simulink model "case9"  (R2024b)
settings: Solver=FixedStepAuto  StartTime=0  StopTime=1  FixedStep=1e-7  RelTol=1e-3
values from neighbouring files (symbols this model uses):
  SG_D_1_D = 0.01056    [IEEE9_case_parameters.m]    (also in case1_parameters.m; case2_parameters.m; case3_parameters.m; case4_parameters.m)
  SG_D_1_EnableSaturation = 0    [IEEE9_case_parameters.m]    (also in case1_parameters.m; case2_parameters.m; case3_parameters.m; case4_parameters.m)
  SG_D_1_f0 = 60    [IEEE9_case_parameters.m]    (also in case1_parameters.m; case2_parameters.m; case3_parameters.m; case4_parameters.m)
  SG_D_1_H = 7.5    [IEEE9_case_parameters.m]    (also in case1_parameters.m; case2_parameters.m; case3_parameters.m; case4_parameters.m)
  SG_D_1_K_A = 20    [IEEE9_case_parameters.m]    (also in case1_parameters.m; case2_parameters.m; case3_parameters.m; case4_parameters.m)
  SG_D_1_K_E = 1.000000e+1    (= 10)    [IEEE9_case_parameters.m]    (also in case1_parameters.m; case2_parameters.m; case3_parameters.m; case4_parameters.m)
  SG_D_1_K_F = 2.363    [IEEE9_case_parameters.m]    (also in case1_parameters.m; case2_parameters.m; case3_parameters.m; case4_parameters.m)
  SG_D_1_K_s = 0.5    [IEEE9_case_parameters.m]    (also in case1_parameters.m = 5; case2_parameters.m = 5; case3_parameters.m = 5; case4_parameters.m = 5)
  SG_D_1_R_a = 0.001088    [IEEE9_case_parameters.m]    (also in case1_parameters.m; case2_parameters.m; case3_parameters.m; case4_parameters.m)
  SG_D_1_S_A = 1    [IEEE9_case_parameters.m]    (also in case1_parameters.m; case2_parameters.m; case3_parameters.m; case4_parameters.m)
  SG_D_1_S_B = 0.103    [IEEE9_case_parameters.m]    (also in case1_parameters.m; case2_parameters.m; case3_parameters.m; case4_parameters.m)
  SG_D_1_S_N = 10.659857    [IEEE9_case_parameters.m]    (also in case1_parameters.m; case2_parameters.m; case3_parameters.m; case4_parameters.m)
  SG_D_1_SpeedPara = 200    [IEEE9_case_parameters.m]    (also in case1_parameters.m; case2_parameters.m; case3_parameters.m; case4_parameters.m)
  SG_D_1_T_0 = 0.720173    [IEEE9_case_parameters.m]    (also in case1_parameters.m = 0.755522; case2_parameters.m = 0.808931; case3_parameters.m = 0.869402; case4_parameters.m = 0.729316)
  SG_D_1_T_1 = 0.3    [IEEE9_case_parameters.m]    (also in case1_parameters.m; case2_parameters.m; case3_parameters.m; case4_parameters.m)
  SG_D_1_T_2 = 0.05    [IEEE9_case_parameters.m]    (also in case1_parameters.m; case2_parameters.m; case3_parameters.m; case4_parameters.m)
  SG_D_1_T_3 = 0.02    [IEEE9_case_parameters.m]    (also in case1_parameters.m; case2_parameters.m; case3_parameters.m; case4_parameters.m)
  SG_D_1_T_4 = 0.005    [IEEE9_case_parameters.m]    (also in case1_parameters.m; case2_parameters.m; case3_parameters.m; case4_parameters.m)
  SG_D_1_T_A = 0.02    [IEEE9_case_parameters.m]    (also in case1_parameters.m; case2_parameters.m; case3_parameters.m; case4_parameters.m)
  SG_D_1_T_dd = 8.000000e+0    (= 8)    [IEEE9_case_parameters.m]    (also in case1_parameters.m; case2_parameters.m; case3_parameters.m; case4_parameters.m)
  SG_D_1_T_ddd = 0.04    [IEEE9_case_parameters.m]    (also in case1_parameters.m; case2_parameters.m; case3_parameters.m; case4_parameters.m)
  SG_D_1_T_E = 0.314    [IEEE9_case_parameters.m]    (also in case1_parameters.m; case2_parameters.m; case3_parameters.m; case4_parameters.m)
  SG_D_1_T_F = 0.35    [IEEE9_case_parameters.m]    (also in case1_parameters.m; case2_parameters.m; case3_parameters.m; case4_parameters.m)
  SG_D_1_T_qd = 0.8    [IEEE9_case_parameters.m]    (also in case1_parameters.m; case2_parameters.m; case3_parameters.m; case4_parameters.m)
  SG_D_1_T_qdd = 0.02    [IEEE9_case_parameters.m]    (also in case1_parameters.m; case2_parameters.m; case3_parameters.m; case4_parameters.m)
  SG_D_1_T_speed = 0.1    [IEEE9_case_parameters.m]    (also in case1_parameters.m = 200; case2_parameters.m = 200; case3_parameters.m = 200; case4_parameters.m = 200)
  SG_D_1_T_w = 0.5    [IEEE9_case_parameters.m]    (also in case1_parameters.m; case2_parameters.m; case3_parameters.m; case4_parameters.m)
  SG_D_1_V_ref = 1.990276    [IEEE9_case_parameters.m]    (also in case1_parameters.m = 2.042296; case2_parameters.m = 2.051388; case3_parameters.m = 2.089584; case4_parameters.m = 2.01845)
  SG_D_1_w_ref = 376.991118    [IEEE9_case_parameters.m]    (also in case1_parameters.m; case2_parameters.m; case3_parameters.m; case4_parameters.m)
  SG_D_1_wb = 6.000000e+1    (= 60)    [IEEE9_case_parameters.m]    (also in case1_parameters.m; case2_parameters.m; case3_parameters.m; case4_parameters.m)
  SG_D_1_x_d = 1.9    [IEEE9_case_parameters.m]    (also in case1_parameters.m; case2_parameters.m; case3_parameters.m; case4_parameters.m)
  SG_D_1_x_dd = 0.302    [IEEE9_case_parameters.m]    (also in case1_parameters.m; case2_parameters.m; case3_parameters.m; case4_parameters.m)
  SG_D_1_x_ddd = 0.204    [IEEE9_case_parameters.m]    (also in case1_parameters.m; case2_parameters.m; case3_parameters.m; case4_parameters.m)
  SG_D_1_x_l = 0.05    [IEEE9_case_parameters.m]    (also in case1_parameters.m; case2_parameters.m; case3_parameters.m; case4_parameters.m)
  SG_D_1_x_q = 1.3    [IEEE9_case_parameters.m]    (also in case1_parameters.m; case2_parameters.m; case3_parameters.m; case4_parameters.m)
  SG_D_1_x_qd = 0.5    [IEEE9_case_parameters.m]    (also in case1_parameters.m; case2_parameters.m; case3_parameters.m; case4_parameters.m)
  SG_D_1_x_qdd = 0.3    [IEEE9_case_parameters.m]    (also in case1_parameters.m; case2_parameters.m; case3_parameters.m; case4_parameters.m)
  SG_D_2_D = 0.02    [IEEE9_case_parameters.m]    (also in case1_parameters.m; case2_parameters.m; case3_parameters.m; case4_parameters.m)
  SG_D_2_EnableSaturation = 0    [IEEE9_case_parameters.m]    (also in case1_parameters.m; case2_parameters.m; case3_parameters.m; case4_parameters.m)
  SG_D_2_f0 = 60    [IEEE9_case_parameters.m]    (also in case1_parameters.m; case2_parameters.m; case3_parameters.m; case4_parameters.m)
  SG_D_2_H = 8.000000e+0    (= 8)    [IEEE9_case_parameters.m]    (also in case1_parameters.m; case2_parameters.m; case3_parameters.m; case4_parameters.m)
  SG_D_2_K_A = 20    [IEEE9_case_parameters.m]    (also in case1_parameters.m; case2_parameters.m; case3_parameters.m; case4_parameters.m)
  SG_D_2_K_E = 1.000000e+1    (= 10)    [IEEE9_case_parameters.m]    (also in case1_parameters.m; case2_parameters.m; case3_parameters.m; case4_parameters.m)
  SG_D_2_K_F = 2.363    [IEEE9_case_parameters.m]    (also in case1_parameters.m; case2_parameters.m; case3_parameters.m; case4_parameters.m)
  SG_D_2_K_s = 0.5    [IEEE9_case_parameters.m]    (also in case1_parameters.m = 4; case2_parameters.m = 4; case3_parameters.m = 4; case4_parameters.m = 4)
  SG_D_2_R_a = 0.001088    [IEEE9_case_parameters.m]    (also in case1_parameters.m; case2_parameters.m; case3_parameters.m; case4_parameters.m)
  SG_D_2_S_A = 1    [IEEE9_case_parameters.m]    (also in case1_parameters.m; case2_parameters.m; case3_parameters.m; case4_parameters.m)
  SG_D_2_S_B = 0.103    [IEEE9_case_parameters.m]    (also in case1_parameters.m; case2_parameters.m; case3_parameters.m; case4_parameters.m)
  SG_D_2_S_N = 10.659857    [IEEE9_case_parameters.m]    (also in case1_parameters.m; case2_parameters.m; case3_parameters.m; case4_parameters.m)
  SG_D_2_SpeedPara = 200    [IEEE9_case_parameters.m]    (also in case1_parameters.m; case2_parameters.m; case3_parameters.m; case4_parameters.m)
  SG_D_2_T_0 = 1.632913    [IEEE9_case_parameters.m]    (also in case1_parameters.m = 1.632925; case2_parameters.m = 1.632915; case3_parameters.m = 1.632914; case4_parameters.m = 1.632927)
  SG_D_2_T_1 = 0.2    [IEEE9_case_parameters.m]    (also in case1_parameters.m; case2_parameters.m; case3_parameters.m; case4_parameters.m)
  SG_D_2_T_2 = 0.05    [IEEE9_case_parameters.m]    (also in case1_parameters.m; case2_parameters.m; case3_parameters.m; case4_parameters.m)
  SG_D_2_T_3 = 0.02    [IEEE9_case_parameters.m]    (also in case1_parameters.m; case2_parameters.m; case3_parameters.m; case4_parameters.m)
  SG_D_2_T_4 = 0.005    [IEEE9_case_parameters.m]    (also in case1_parameters.m; case2_parameters.m; case3_parameters.m; case4_parameters.m)
  SG_D_2_T_A = 0.02    [IEEE9_case_parameters.m]    (also in case1_parameters.m; case2_parameters.m; case3_parameters.m; case4_parameters.m)
  SG_D_2_T_dd = 7.9    [IEEE9_case_parameters.m]    (also in case1_parameters.m; case2_parameters.m; case3_parameters.m; case4_parameters.m)
  SG_D_2_T_ddd = 0.04    [IEEE9_case_parameters.m]    (also in case1_parameters.m; case2_parameters.m; case3_parameters.m; case4_parameters.m)
  SG_D_2_T_E = 0.314    [IEEE9_case_parameters.m]    (also in case1_parameters.m; case2_parameters.m; case3_parameters.m; case4_parameters.m)
  SG_D_2_T_F = 0.35    [IEEE9_case_parameters.m]    (also in case1_parameters.m; case2_parameters.m; case3_parameters.m; case4_parameters.m)
  SG_D_2_T_qd = 0.8    [IEEE9_case_parameters.m]    (also in case1_parameters.m; case2_parameters.m; case3_parameters.m; case4_parameters.m)
  SG_D_2_T_qdd = 0.015    [IEEE9_case_parameters.m]    (also in case1_parameters.m; case2_parameters.m; case3_parameters.m; case4_parameters.m)
  SG_D_2_T_speed = 0.1    [IEEE9_case_parameters.m]    (also in case1_parameters.m = 150; case2_parameters.m = 150; case3_parameters.m = 150; case4_parameters.m = 150)
  SG_D_2_T_w = 0.35    [IEEE9_case_parameters.m]    (also in case1_parameters.m; case2_parameters.m; case3_parameters.m; case4_parameters.m)
  SG_D_2_V_ref = 2.58547    [IEEE9_case_parameters.m]    (also in case1_parameters.m = 2.597896; case2_parameters.m = 2.587136; case3_parameters.m = 2.586042; case4_parameters.m = 2.599679)
  SG_D_2_w_ref = 376.991118    [IEEE9_case_parameters.m]    (also in case1_parameters.m; case2_parameters.m; case3_parameters.m; case4_parameters.m)
  SG_D_2_wb = 6.000000e+1    (= 60)    [IEEE9_case_parameters.m]    (also in case1_parameters.m; case2_parameters.m; case3_parameters.m; case4_parameters.m)
  SG_D_2_x_d = 1.8    [IEEE9_case_parameters.m]    (also in case1_parameters.m; case2_parameters.m; case3_parameters.m; case4_parameters.m)
  SG_D_2_x_dd = 0.302    [IEEE9_case_parameters.m]    (also in case1_parameters.m; case2_parameters.m; case3_parameters.m; case4_parameters.m)
  SG_D_2_x_ddd = 0.204    [IEEE9_case_parameters.m]    (also in case1_parameters.m; case2_parameters.m; case3_parameters.m; case4_parameters.m)
  SG_D_2_x_l = 0.05    [IEEE9_case_parameters.m]    (also in case1_parameters.m; case2_parameters.m; case3_parameters.m; case4_parameters.m)
  SG_D_2_x_q = 1.25    [IEEE9_case_parameters.m]    (also in case1_parameters.m; case2_parameters.m; case3_parameters.m; case4_parameters.m)
  SG_D_2_x_qd = 0.5    [IEEE9_case_parameters.m]    (also in case1_parameters.m; case2_parameters.m; case3_parameters.m; case4_parameters.m)
  SG_D_2_x_qdd = 0.3    [IEEE9_case_parameters.m]    (also in case1_parameters.m; case2_parameters.m; case3_parameters.m; case4_parameters.m)
  SG_D_3_D = 0.02    [IEEE9_case_parameters.m]    (also in case1_parameters.m; case2_parameters.m; case3_parameters.m; case4_parameters.m)
  SG_D_3_EnableSaturation = 0    [IEEE9_case_parameters.m]    (also in case1_parameters.m; case2_parameters.m; case3_parameters.m; case4_parameters.m)
  SG_D_3_f0 = 60    [IEEE9_case_parameters.m]    (also in case1_parameters.m; case2_parameters.m; case3_parameters.m; case4_parameters.m)
  SG_D_3_H = 7.7    [IEEE9_case_parameters.m]    (also in case1_parameters.m; case2_parameters.m; case3_parameters.m; case4_parameters.m)
  SG_D_3_K_A = 20    [IEEE9_case_parameters.m]    (also in case1_parameters.m; case2_parameters.m; case3_parameters.m; case4_parameters.m)
  SG_D_3_K_E = 1.000000e+1    (= 10)    [IEEE9_case_parameters.m]    (also in case1_parameters.m; case2_parameters.m; case3_parameters.m; case4_parameters.m)
  SG_D_3_K_F = 2.363    [IEEE9_case_parameters.m]    (also in case1_parameters.m; case2_parameters.m; case3_parameters.m; case4_parameters.m)
  SG_D_3_K_s = 0.2    [IEEE9_case_parameters.m]    (also in case1_parameters.m = 2; case2_parameters.m = 2; case3_parameters.m = 2; case4_parameters.m = 2)
  SG_D_3_R_a = 0.001088    [IEEE9_case_parameters.m]    (also in case1_parameters.m; case2_parameters.m; case3_parameters.m; case4_parameters.m)
  SG_D_3_S_A = 1    [IEEE9_case_parameters.m]    (also in case1_parameters.m; case2_parameters.m; case3_parameters.m; case4_parameters.m)
  SG_D_3_S_B = 0.103    [IEEE9_case_parameters.m]    (also in case1_parameters.m; case2_parameters.m; case3_parameters.m; case4_parameters.m)
  SG_D_3_S_N = 10.659857    [IEEE9_case_parameters.m]    (also in case1_parameters.m; case2_parameters.m; case3_parameters.m; case4_parameters.m)
  SG_D_3_SpeedPara = 200    [IEEE9_case_parameters.m]    (also in case1_parameters.m; case2_parameters.m; case3_parameters.m; case4_parameters.m)
  SG_D_3_T_0 = 0.850788    [IEEE9_case_parameters.m]    (also in case1_parameters.m = 0.850786; case2_parameters.m = 0.850787; case3_parameters.m; case4_parameters.m = 0.850786)
  SG_D_3_T_1 = 0.2    [IEEE9_case_parameters.m]    (also in case1_parameters.m; case2_parameters.m; case3_parameters.m; case4_parameters.m)
  SG_D_3_T_2 = 0.05    [IEEE9_case_parameters.m]    (also in case1_parameters.m; case2_parameters.m; case3_parameters.m; case4_parameters.m)
  SG_D_3_T_3 = 0.02    [IEEE9_case_parameters.m]    (also in case1_parameters.m; case2_parameters.m; case3_parameters.m; case4_parameters.m)
  SG_D_3_T_4 = 0.005    [IEEE9_case_parameters.m]    (also in case1_parameters.m; case2_parameters.m; case3_parameters.m; case4_parameters.m)
  SG_D_3_T_A = 0.02    [IEEE9_case_parameters.m]    (also in case1_parameters.m; case2_parameters.m; case3_parameters.m; case4_parameters.m)
  SG_D_3_T_dd = 8.1    [IEEE9_case_parameters.m]    (also in case1_parameters.m; case2_parameters.m; case3_parameters.m; case4_parameters.m)
  SG_D_3_T_ddd = 0.04    [IEEE9_case_parameters.m]    (also in case1_parameters.m; case2_parameters.m; case3_parameters.m; case4_parameters.m)
  SG_D_3_T_E = 0.314    [IEEE9_case_parameters.m]    (also in case1_parameters.m; case2_parameters.m; case3_parameters.m; case4_parameters.m)
  SG_D_3_T_F = 0.35    [IEEE9_case_parameters.m]    (also in case1_parameters.m; case2_parameters.m; case3_parameters.m; case4_parameters.m)
  SG_D_3_T_qd = 0.8    [IEEE9_case_parameters.m]    (also in case1_parameters.m; case2_parameters.m; case3_parameters.m; case4_parameters.m)
  SG_D_3_T_qdd = 0.015    [IEEE9_case_parameters.m]    (also in case1_parameters.m; case2_parameters.m; case3_parameters.m; case4_parameters.m)
  SG_D_3_T_speed = 0.1    [IEEE9_case_parameters.m]    (also in case1_parameters.m = 180; case2_parameters.m = 180; case3_parameters.m = 180; case4_parameters.m = 180)
  SG_D_3_T_w = 0.4    [IEEE9_case_parameters.m]    (also in case1_parameters.m; case2_parameters.m; case3_parameters.m; case4_parameters.m)
  SG_D_3_V_ref = 1.892727    [IEEE9_case_parameters.m]    (also in case1_parameters.m = 1.906439; case2_parameters.m = 1.895535; case3_parameters.m = 1.892105; case4_parameters.m = 1.906598)
  SG_D_3_w_ref = 376.991118    [IEEE9_case_parameters.m]    (also in case1_parameters.m; case2_parameters.m; case3_parameters.m; case4_parameters.m)
  SG_D_3_wb = 6.000000e+1    (= 60)    [IEEE9_case_parameters.m]    (also in case1_parameters.m; case2_parameters.m; case3_parameters.m; case4_parameters.m)
  SG_D_3_x_d = 1.85    [IEEE9_case_parameters.m]    (also in case1_parameters.m; case2_parameters.m; case3_parameters.m; case4_parameters.m)
  SG_D_3_x_dd = 0.302    [IEEE9_case_parameters.m]    (also in case1_parameters.m; case2_parameters.m; case3_parameters.m; case4_parameters.m)
  SG_D_3_x_ddd = 0.204    [IEEE9_case_parameters.m]    (also in case1_parameters.m; case2_parameters.m; case3_parameters.m; case4_parameters.m)
  SG_D_3_x_l = 0.05    [IEEE9_case_parameters.m]    (also in case1_parameters.m; case2_parameters.m; case3_parameters.m; case4_parameters.m)
  SG_D_3_x_q = 1.2    [IEEE9_case_parameters.m]    (also in case1_parameters.m; case2_parameters.m; case3_parameters.m; case4_parameters.m)
  SG_D_3_x_qd = 0.5    [IEEE9_case_parameters.m]    (also in case1_parameters.m; case2_parameters.m; case3_parameters.m; case4_parameters.m)
  SG_D_3_x_qdd = 0.3    [IEEE9_case_parameters.m]    (also in case1_parameters.m; case2_parameters.m; case3_parameters.m; case4_parameters.m)
(part 9 of 12)

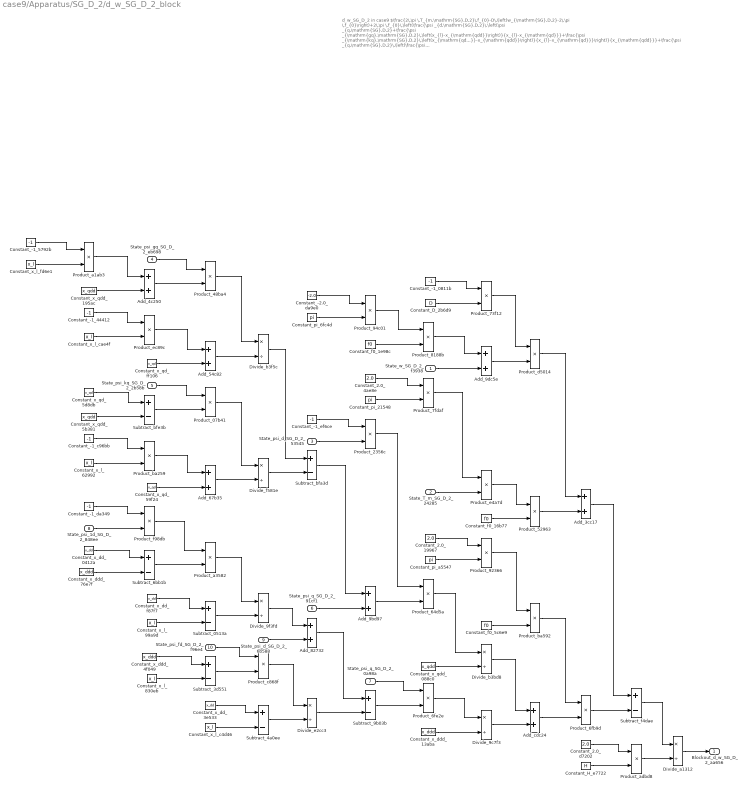
== system case9/Apparatus/SG_D_2/d_w_SG_D_2_block ==
  note: d_w_SG_D_2 in case9
      | $\frac{2\,\pi \,T_{m,\mathrm{SG},D,2}\,f_{0}-D\,\left(w_{\mathrm{SG},D,2}-2\,\pi \,f_{0}\right)+2\,\pi \,f_{0}\,\left(\frac{\psi _{d,\mathrm{SG},D,2}\,\left(\psi _{q,\mathrm{SG},D,2}+\frac{\psi _{\mathrm{gq},\mathrm{SG},D,2}\,\left(x_{l}-x_{\mathrm{qdd}}\right)}{x_{l}-x_{\mathrm{qd}}}+\frac{\psi _{\mathrm{kq},\mathrm{SG},D,2}\,\left(x_{\mathrm{qd}}-x_{\mathrm{qdd}}\right)}{x_{l}-x_{\mathrm{qd}}}\right)}{x_{\mathrm{qdd}}}+\frac{\psi _{q,\mathrm{SG},D,2}\,\left(\frac{\psi _{\mathrm{1d},\mathrm{SG},D,2}\,\left(x_{\mathrm{dd}}-x_{\mathrm{ddd}}\right)}{x_{\mathrm{dd}}-x_{l}}-\psi _{d,\mathrm{SG},D,2}+\frac{\psi _{\mathrm{fd},\mathrm{SG},D,2}\,\left(x_{\mathrm{ddd}}-x_{l}\right)}{x_{\mathrm{dd}}-x_{l}}\right)}{x_{\mathrm{ddd}}}\right)}{2\,H}$
      | Automatically generated on 2025-10-31 19:35:00 .
  State_w_SG_D_2_f3938 : Inport
  State_T_m_SG_D_2_24285 : Inport  Port=2
  State_psi_d_SG_D_2_53545 : Inport  Port=3
  State_psi_gq_SG_D_2_eb698 : Inport  Port=4
  State_psi_kq_SG_D_2_2b58b : Inport  Port=5
  State_psi_q_SG_D_2_91cf1 : Inport  Port=6
  State_psi_q_SG_D_2_0a98a : Inport  Port=7
  State_psi_1d_SG_D_2_848ee : Inport  Port=8
  State_psi_d_SG_D_2_6b588 : Inport  Port=9
  State_psi_fd_SG_D_2_f96e4 : Inport  Port=10
  Add_3cc17 : Sum
  Add_4c250 : Sum
  Add_54c82 : Sum
  Add_67b35 : Sum
  Add_82732 : Sum
  Add_9bd97 : Sum
  Add_9dc5e : Sum
  Add_cdc24 : Sum
  Constant_-1_0811b : Constant  Value=-1
  Constant_-1_44412 : Constant  Value=-1
  Constant_-1_5792b : Constant  Value=-1
  Constant_-1_c96bb : Constant  Value=-1
  Constant_-1_da349 : Constant  Value=-1
  Constant_-1_ef6ce : Constant  Value=-1
  Constant_-2.0_da9e0 : Constant  Value=-2.0
  Constant_2.0_19967 : Constant  Value=2.0
  Constant_2.0_4ae8e : Constant  Value=2.0
  Constant_2.0_d7202 : Constant  Value=2.0
  Constant_D_2b6d9 : Constant  Value=D
  Constant_H_e7722 : Constant  Value=H
  Constant_f0_16b77 : Constant  Value=f0
  Constant_f0_1e98c : Constant  Value=f0
  Constant_f0_5c6e9 : Constant  Value=f0
  Constant_pi_21548 : Constant  Value=pi
  Constant_pi_6fc4d : Constant  Value=pi
  Constant_pi_a5547 : Constant  Value=pi
  Constant_x_dd_0412a : Constant  Value=x_dd
  Constant_x_dd_3e533 : Constant  Value=x_dd
  Constant_x_dd_f87f7 : Constant  Value=x_dd
  Constant_x_ddd_13aba : Constant  Value=x_ddd
  Constant_x_ddd_4f049 : Constant  Value=x_ddd
  Constant_x_ddd_76e7f : Constant  Value=x_ddd
  Constant_x_l_62992 : Constant  Value=x_l
  Constant_x_l_830eb : Constant  Value=x_l
  Constant_x_l_99a9d : Constant  Value=x_l
  Constant_x_l_c4d46 : Constant  Value=x_l
  Constant_x_l_cae4f : Constant  Value=x_l
  Constant_x_l_fd6e1 : Constant  Value=x_l
  Constant_x_qd_59f24 : Constant  Value=x_qd
  Constant_x_qd_5d8db : Constant  Value=x_qd
  Constant_x_qd_ff106 : Constant  Value=x_qd
  Constant_x_qdd_088c0 : Constant  Value=x_qdd
  Constant_x_qdd_195ac : Constant  Value=x_qdd
  Constant_x_qdd_5b381 : Constant  Value=x_qdd
  Divide_9c7f3 : Product  Inputs=*/
  Divide_9f3fd : Product  Inputs=*/
  Divide_a1312 : Product  Inputs=*/
  Divide_b3bd8 : Product  Inputs=*/
  Divide_b3f5c : Product  Inputs=*/
  Divide_e2cc3 : Product  Inputs=*/
  Divide_f581e : Product  Inputs=*/
  Product_07b41 : Product
  Product_2356c : Product
  Product_48ba4 : Product
  Product_52963 : Product
  Product_64d5a : Product
  Product_6fb9d : Product
  Product_6fe2e : Product
  Product_73f12 : Product
  Product_7fdaf : Product
  Product_8188b : Product
  Product_92366 : Product
  Product_94c01 : Product
  Product_a1ab3 : Product
  Product_a3582 : Product
  Product_adbd8 : Product
  Product_ba259 : Product
  Product_ba592 : Product
  Product_c868f : Product
  Product_d5014 : Product
  Product_e4a7d : Product
  Product_ec89c : Product
  Product_f98db : Product
  Subtract_0513a : Sum  Inputs=+-
  Subtract_3d551 : Sum  Inputs=+-
  Subtract_4a0ee : Sum  Inputs=+-
  Subtract_6bb1b : Sum  Inputs=+-
  Subtract_9b03b : Sum  Inputs=+-
  Subtract_bfa3d : Sum  Inputs=+-
  Subtract_bfe3b : Sum  Inputs=+-
  Subtract_f4dae : Sum  Inputs=+-
  Blockout_d_w_SG_D_2_aa656 : Outport
  wires:
  Constant_x_qd_5d8db/1 -> Subtract_bfe3b/1
  Constant_-1_c96bb/1 -> Product_ba259/1
  Constant_-1_5792b/1 -> Product_a1ab3/1
  Constant_x_qdd_5b381/1 -> Subtract_bfe3b/2
  Subtract_4a0ee/1 -> Divide_e2cc3/2
  Constant_x_l_62992/1 -> Product_ba259/2
  Constant_x_l_fd6e1/1 -> Product_a1ab3/2
  Product_ba259/1 -> Add_67b35/1
  Product_a1ab3/1 -> Add_4c250/1
  Constant_x_l_99a9d/1 -> Subtract_0513a/2
  Constant_x_l_cae4f/1 -> Product_ec89c/2
  Constant_x_ddd_13aba/1 -> Divide_9c7f3/2
  Subtract_3d551/1 -> Product_c868f/2
  Constant_x_qd_59f24/1 -> Add_67b35/2
  Constant_x_qdd_195ac/1 -> Add_4c250/2
  Constant_-1_44412/1 -> Product_ec89c/1
  State_psi_d_SG_D_2_53545/1 -> Product_2356c/2
  Constant_-1_da349/1 -> Product_f98db/1
  State_w_SG_D_2_f3938/1 -> Add_9dc5e/2
  Product_ec89c/1 -> Add_54c82/1
  State_psi_1d_SG_D_2_848ee/1 -> Product_f98db/2
  Constant_x_dd_0412a/1 -> Subtract_6bb1b/1
  Divide_b3f5c/1 -> Subtract_bfa3d/1
  Subtract_bfe3b/1 -> Product_07b41/2
  Constant_x_ddd_76e7f/1 -> Subtract_6bb1b/2
  State_psi_gq_SG_D_2_eb698/1 -> Product_48ba4/1
  Add_67b35/1 -> Divide_f581e/2
  State_psi_d_SG_D_2_6b588/1 -> Add_82732/2
  Add_4c250/1 -> Product_48ba4/2
  Constant_x_qd_ff106/1 -> Add_54c82/2
  State_psi_kq_SG_D_2_2b58b/1 -> Product_07b41/1
  Product_f98db/1 -> Product_a3582/1
  Subtract_6bb1b/1 -> Product_a3582/2
  Constant_pi_21548/1 -> Product_7fdaf/2
  Constant_x_dd_f87f7/1 -> Subtract_0513a/1
  Constant_x_ddd_4f049/1 -> Subtract_3d551/1
  Constant_x_l_830eb/1 -> Subtract_3d551/2
  Product_48ba4/1 -> Divide_b3f5c/1
  Add_54c82/1 -> Divide_b3f5c/2
  Add_9bd97/1 -> Product_64d5a/2
  Product_07b41/1 -> Divide_f581e/1
  Constant_pi_6fc4d/1 -> Product_94c01/2
  Product_a3582/1 -> Divide_9f3fd/1
  Subtract_0513a/1 -> Divide_9f3fd/2
  State_psi_fd_SG_D_2_f96e4/1 -> Product_c868f/1
  Divide_9f3fd/1 -> Add_82732/1
  Constant_x_dd_3e533/1 -> Subtract_4a0ee/1
  Constant_x_l_c4d46/1 -> Subtract_4a0ee/2
  Divide_f581e/1 -> Subtract_bfa3d/2
  Product_c868f/1 -> Divide_e2cc3/1
  Constant_-1_ef6ce/1 -> Product_2356c/1
  Constant_-2.0_da9e0/1 -> Product_94c01/1
  Subtract_bfa3d/1 -> Add_9bd97/1
  Subtract_9b03b/1 -> Product_6fe2e/2
  State_psi_q_SG_D_2_91cf1/1 -> Add_9bd97/2
  Constant_D_2b6d9/1 -> Product_73f12/2
  Add_82732/1 -> Subtract_9b03b/1
  Divide_e2cc3/1 -> Subtract_9b03b/2
  Product_94c01/1 -> Product_8188b/1
  Constant_f0_1e98c/1 -> Product_8188b/2
  Constant_2.0_4ae8e/1 -> Product_7fdaf/1
  Product_2356c/1 -> Product_64d5a/1
  State_psi_q_SG_D_2_0a98a/1 -> Product_6fe2e/1
  Constant_-1_0811b/1 -> Product_73f12/1
  Product_8188b/1 -> Add_9dc5e/1
  Product_7fdaf/1 -> Product_e4a7d/1
  State_T_m_SG_D_2_24285/1 -> Product_e4a7d/2
  Constant_2.0_19967/1 -> Product_92366/1
  Constant_pi_a5547/1 -> Product_92366/2
  Product_64d5a/1 -> Divide_b3bd8/1
  Constant_x_qdd_088c0/1 -> Divide_b3bd8/2
  Product_6fe2e/1 -> Divide_9c7f3/1
  Product_73f12/1 -> Product_d5014/1
  Add_9dc5e/1 -> Product_d5014/2
  Product_e4a7d/1 -> Product_52963/1
  Constant_f0_16b77/1 -> Product_52963/2
  Product_92366/1 -> Product_ba592/1
  Constant_f0_5c6e9/1 -> Product_ba592/2
  Divide_b3bd8/1 -> Add_cdc24/1
  Divide_9c7f3/1 -> Add_cdc24/2
  Product_d5014/1 -> Add_3cc17/1
  Product_52963/1 -> Add_3cc17/2
  Product_ba592/1 -> Product_6fb9d/1
  Add_cdc24/1 -> Product_6fb9d/2
  Add_3cc17/1 -> Subtract_f4dae/1
  Product_6fb9d/1 -> Subtract_f4dae/2
  Constant_2.0_d7202/1 -> Product_adbd8/1
  Constant_H_e7722/1 -> Product_adbd8/2
  Subtract_f4dae/1 -> Divide_a1312/1
  Product_adbd8/1 -> Divide_a1312/2
  Divide_a1312/1 -> Blockout_d_w_SG_D_2_aa656/1

== system case9/Apparatus/SG_D_2/i_d_SG_D_2_block ==
  note: i_d_SG_D_2 in case9
      | $\frac{\sin\left(\theta _{\mathrm{SG},D,2}\right)\,\left(\frac{\psi _{\mathrm{1d},\mathrm{SG},D,2}\,\left(x_{\mathrm{dd}}-x_{\mathrm{ddd}}\right)}{x_{\mathrm{dd}}-x_{l}}-\psi _{d,\mathrm{SG},D,2}+\frac{\psi _{\mathrm{fd},\mathrm{SG},D,2}\,\left(x_{\mathrm{ddd}}-x_{l}\right)}{x_{\mathrm{dd}}-x_{l}}\right)}{x_{\mathrm{ddd}}}-\frac{\cos\left(\theta _{\mathrm{SG},D,2}\right)\,\left(\psi _{q,\mathrm{SG},D,2}+\frac{\psi _{\mathrm{gq},\mathrm{SG},D,2}\,\left(x_{l}-x_{\mathrm{qdd}}\right)}{x_{l}-x_{\mathrm{qd}}}+\frac{\psi _{\mathrm{kq},\mathrm{SG},D,2}\,\left(x_{\mathrm{qd}}-x_{\mathrm{qdd}}\right)}{x_{l}-x_{\mathrm{qd}}}\right)}{x_{\mathrm{qdd}}}$
      | Automatically generated on 2025-10-31 19:35:06 .
  State_psi_gq_SG_D_2_4662b : Inport
  State_psi_kq_SG_D_2_698d0 : Inport  Port=2
  State_psi_q_SG_D_2_36cd5 : Inport  Port=3
  State_theta_SG_D_2_40ee4 : Inport  Port=4
  State_psi_1d_SG_D_2_a2f3b : Inport  Port=5
  State_psi_d_SG_D_2_56fc9 : Inport  Port=6
  State_psi_fd_SG_D_2_81fbd : Inport  Port=7
  State_theta_SG_D_2_40f5f : Inport  Port=8
  Add_3334b : Sum
  Add_906bd : Sum
  Add_a5c99 : Sum
  Add_b6380 : Sum
  Add_e77ea : Sum
  Constant_-1_237f5 : Constant  Value=-1
  Constant_-1_99fb6 : Constant  Value=-1
  Constant_-1_b5e39 : Constant  Value=-1
  Constant_-1_ba0b3 : Constant  Value=-1
  Constant_-1_e4820 : Constant  Value=-1
  Constant_x_dd_10e98 : Constant  Value=x_dd
  Constant_x_dd_565cc : Constant  Value=x_dd
  Constant_x_dd_e6095 : Constant  Value=x_dd
  Constant_x_ddd_015a1 : Constant  Value=x_ddd
  Constant_x_ddd_399a2 : Constant  Value=x_ddd
  Constant_x_ddd_740f4 : Constant  Value=x_ddd
  Constant_x_l_13a33 : Constant  Value=x_l
  Constant_x_l_5a17f : Constant  Value=x_l
  Constant_x_l_70936 : Constant  Value=x_l
  Constant_x_l_8d494 : Constant  Value=x_l
  Constant_x_l_93f95 : Constant  Value=x_l
  Constant_x_l_a8278 : Constant  Value=x_l
  Constant_x_qd_0d6a6 : Constant  Value=x_qd
  Constant_x_qd_75f2f : Constant  Value=x_qd
  Constant_x_qd_f1c45 : Constant  Value=x_qd
  Constant_x_qdd_c1732 : Constant  Value=x_qdd
  Constant_x_qdd_d22ec : Constant  Value=x_qdd
  Constant_x_qdd_ded7a : Constant  Value=x_qdd
  Divide_13a6c : Product  Inputs=*/
  Divide_60d19 : Product  Inputs=*/
  Divide_710e2 : Product  Inputs=*/
  Divide_8690d : Product  Inputs=*/
  Divide_94831 : Product  Inputs=*/
  Divide_ed957 : Product  Inputs=*/
  MathFunc_cos_65f0c : Trigonometry  Operator=cos
  MathFunc_sin_6cf7a : Trigonometry
  Product_1d520 : Product
  Product_2ab91 : Product
  Product_3af98 : Product
  Product_48c05 : Product
  Product_5a91d : Product
  Product_92bbc : Product
  Product_a866b : Product
  Product_abbff : Product
  Product_ccc27 : Product
  Product_eb74b : Product
  Product_f3706 : Product
  Subtract_0a275 : Sum  Inputs=+-
  Subtract_0f5dd : Sum  Inputs=+-
  Subtract_1282d : Sum  Inputs=+-
  Subtract_17892 : Sum  Inputs=+-
  Subtract_1a32d : Sum  Inputs=+-
  Subtract_3ebd0 : Sum  Inputs=+-
  Subtract_510f6 : Sum  Inputs=+-
  Subtract_d118c : Sum  Inputs=+-
  Blockout_i_d_SG_D_2_11970 : Outport
  wires:
  Constant_x_ddd_399a2/1 -> Subtract_1282d/1
  Constant_x_qd_75f2f/1 -> Subtract_d118c/1
  Constant_-1_99fb6/1 -> Product_ccc27/1
  Constant_-1_b5e39/1 -> Product_a866b/1
  Subtract_510f6/1 -> Blockout_i_d_SG_D_2_11970/1
  Constant_x_qdd_ded7a/1 -> Subtract_d118c/2
  Constant_x_l_8d494/1 -> Product_ccc27/2
  Constant_x_l_93f95/1 -> Product_a866b/2
  Product_ccc27/1 -> Add_e77ea/1
  Product_a866b/1 -> Add_b6380/1
  Constant_x_l_5a17f/1 -> Product_3af98/2
  Constant_x_qd_0d6a6/1 -> Add_e77ea/2
  Constant_x_qdd_d22ec/1 -> Add_b6380/2
  Constant_x_qdd_c1732/1 -> Divide_94831/2
  MathFunc_cos_65f0c/1 -> Product_48c05/2
  Constant_-1_237f5/1 -> Product_3af98/1
  State_psi_gq_SG_D_2_4662b/1 -> Product_92bbc/1
  Subtract_1282d/1 -> Product_abbff/2
  Product_eb74b/1 -> Product_f3706/1
  Add_e77ea/1 -> Divide_13a6c/2
  Add_b6380/1 -> Product_92bbc/2
  Product_abbff/1 -> Divide_710e2/1
  Product_3af98/1 -> Add_a5c99/1
  Constant_x_qd_f1c45/1 -> Add_a5c99/2
  State_theta_SG_D_2_40f5f/1 -> MathFunc_sin_6cf7a/1
  State_psi_kq_SG_D_2_698d0/1 -> Product_1d520/1
  Add_906bd/1 -> Subtract_0a275/1
  Subtract_d118c/1 -> Product_1d520/2
  Product_92bbc/1 -> Divide_60d19/1
  Constant_-1_ba0b3/1 -> Product_eb74b/1
  State_psi_1d_SG_D_2_a2f3b/1 -> Product_eb74b/2
  State_psi_fd_SG_D_2_81fbd/1 -> Product_abbff/1
  Constant_x_dd_565cc/1 -> Subtract_1a32d/1
  Product_f3706/1 -> Divide_8690d/1
  Constant_x_ddd_740f4/1 -> Subtract_1a32d/2
  Divide_710e2/1 -> Subtract_0a275/2
  Add_a5c99/1 -> Divide_60d19/2
  Product_5a91d/1 -> Divide_ed957/1
  Product_1d520/1 -> Divide_13a6c/1
  Constant_-1_e4820/1 -> Product_2ab91/1
  Subtract_0f5dd/1 -> Divide_710e2/2
  Subtract_1a32d/1 -> Product_f3706/2
  Constant_x_dd_e6095/1 -> Subtract_17892/1
  Subtract_0a275/1 -> Product_5a91d/1
  Constant_x_l_70936/1 -> Subtract_17892/2
  Constant_x_l_a8278/1 -> Subtract_1282d/2
  Divide_60d19/1 -> Subtract_3ebd0/1
  Divide_ed957/1 -> Subtract_510f6/2
  Divide_13a6c/1 -> Subtract_3ebd0/2
  Subtract_17892/1 -> Divide_8690d/2
  Constant_x_dd_10e98/1 -> Subtract_0f5dd/1
  Divide_94831/1 -> Subtract_510f6/1
  Constant_x_l_13a33/1 -> Subtract_0f5dd/2
  Subtract_3ebd0/1 -> Add_3334b/1
  State_psi_q_SG_D_2_36cd5/1 -> Add_3334b/2
  Constant_x_ddd_015a1/1 -> Divide_ed957/2
  MathFunc_sin_6cf7a/1 -> Product_5a91d/2
  Divide_8690d/1 -> Add_906bd/1
  State_psi_d_SG_D_2_56fc9/1 -> Add_906bd/2
  Add_3334b/1 -> Product_2ab91/2
  State_theta_SG_D_2_40ee4/1 -> MathFunc_cos_65f0c/1
  Product_2ab91/1 -> Product_48c05/1
  Product_48c05/1 -> Divide_94831/1

== system case9/Apparatus/SG_D_2/i_q_SG_D_2_block ==
  note: i_q_SG_D_2 in case9
      | $-\frac{\sin\left(\theta _{\mathrm{SG},D,2}\right)\,\left(\psi _{q,\mathrm{SG},D,2}+\frac{\psi _{\mathrm{gq},\mathrm{SG},D,2}\,\left(x_{l}-x_{\mathrm{qdd}}\right)}{x_{l}-x_{\mathrm{qd}}}+\frac{\psi _{\mathrm{kq},\mathrm{SG},D,2}\,\left(x_{\mathrm{qd}}-x_{\mathrm{qdd}}\right)}{x_{l}-x_{\mathrm{qd}}}\right)}{x_{\mathrm{qdd}}}-\frac{\cos\left(\theta _{\mathrm{SG},D,2}\right)\,\left(\frac{\psi _{\mathrm{1d},\mathrm{SG},D,2}\,\left(x_{\mathrm{dd}}-x_{\mathrm{ddd}}\right)}{x_{\mathrm{dd}}-x_{l}}-\psi _{d,\mathrm{SG},D,2}+\frac{\psi _{\mathrm{fd},\mathrm{SG},D,2}\,\left(x_{\mathrm{ddd}}-x_{l}\right)}{x_{\mathrm{dd}}-x_{l}}\right)}{x_{\mathrm{ddd}}}$
      | Automatically generated on 2025-10-31 19:35:07 .
  State_psi_gq_SG_D_2_44a2c : Inport
  State_psi_kq_SG_D_2_69c0a : Inport  Port=2
  State_psi_q_SG_D_2_754c0 : Inport  Port=3
  State_theta_SG_D_2_97c1c : Inport  Port=4
  State_psi_1d_SG_D_2_5fde3 : Inport  Port=5
  State_psi_d_SG_D_2_f9261 : Inport  Port=6
  State_psi_fd_SG_D_2_bd312 : Inport  Port=7
  State_theta_SG_D_2_8f6ba : Inport  Port=8
  Add_3aa3a : Sum
  Add_3ec1d : Sum
  Add_424f6 : Sum
  Add_4dab6 : Sum
  Add_6b69c : Sum
  Add_809c3 : Sum
  Constant_-1_bda3a : Constant  Value=-1
  Constant_-1_be823 : Constant  Value=-1
  Constant_-1_c1860 : Constant  Value=-1
  Constant_-1_d5e2f : Constant  Value=-1
  Constant_-1_ff025 : Constant  Value=-1
  Constant_x_dd_1c1a3 : Constant  Value=x_dd
  Constant_x_dd_4b546 : Constant  Value=x_dd
  Constant_x_dd_7f840 : Constant  Value=x_dd
  Constant_x_ddd_15a6e : Constant  Value=x_ddd
  Constant_x_ddd_8ff67 : Constant  Value=x_ddd
  Constant_x_ddd_b0a16 : Constant  Value=x_ddd
  Constant_x_l_2477e : Constant  Value=x_l
  Constant_x_l_40cc1 : Constant  Value=x_l
  Constant_x_l_4b18d : Constant  Value=x_l
  Constant_x_l_75e55 : Constant  Value=x_l
  Constant_x_l_96a62 : Constant  Value=x_l
  Constant_x_l_b2ff0 : Constant  Value=x_l
  Constant_x_qd_0b95a : Constant  Value=x_qd
  Constant_x_qd_179db : Constant  Value=x_qd
  Constant_x_qd_24ffc : Constant  Value=x_qd
  Constant_x_qdd_100ca : Constant  Value=x_qdd
  Constant_x_qdd_5a495 : Constant  Value=x_qdd
  Constant_x_qdd_d7281 : Constant  Value=x_qdd
  Divide_05d18 : Product  Inputs=*/
  Divide_7c35b : Product  Inputs=*/
  Divide_859a3 : Product  Inputs=*/
  Divide_99946 : Product  Inputs=*/
  Divide_e5b49 : Product  Inputs=*/
  Divide_ffc3b : Product  Inputs=*/
  MathFunc_cos_e8163 : Trigonometry  Operator=cos
  MathFunc_sin_12ad6 : Trigonometry
  Product_1e598 : Product
  Product_3b575 : Product
  Product_67151 : Product
  Product_6aa76 : Product
  Product_6d26f : Product
  Product_7be1b : Product
  Product_80218 : Product
  Product_8602e : Product
  Product_9cdc9 : Product
  Product_ae213 : Product
  Product_f553d : Product
  Subtract_01084 : Sum  Inputs=+-
  Subtract_0f46b : Sum  Inputs=+-
  Subtract_8bd1d : Sum  Inputs=+-
  Subtract_c16dc : Sum  Inputs=+-
  Subtract_cdbd8 : Sum  Inputs=+-
  Subtract_ce231 : Sum  Inputs=+-
  Subtract_efc4f : Sum  Inputs=+-
  Blockout_i_q_SG_D_2_87aea : Outport
  wires:
  MathFunc_sin_12ad6/1 -> Product_6d26f/2
  Product_ae213/1 -> Product_6d26f/1
  Constant_-1_be823/1 -> Product_7be1b/1
  Constant_-1_ff025/1 -> Product_8602e/1
  Constant_x_l_b2ff0/1 -> Product_7be1b/2
  Product_7be1b/1 -> Add_3ec1d/1
  Subtract_0f46b/1 -> Product_3b575/2
  Constant_x_qdd_5a495/1 -> Subtract_efc4f/2
  Constant_x_qdd_d7281/1 -> Add_3ec1d/2
  Add_424f6/1 -> Product_ae213/2
  Constant_x_l_40cc1/1 -> Product_8602e/2
  Constant_x_qd_0b95a/1 -> Subtract_efc4f/1
  Constant_-1_bda3a/1 -> Product_9cdc9/1
  Constant_x_l_75e55/1 -> Product_9cdc9/2
  State_psi_1d_SG_D_2_5fde3/1 -> Product_1e598/2
  State_psi_gq_SG_D_2_44a2c/1 -> Product_67151/1
  Add_3ec1d/1 -> Product_67151/2
  Product_8602e/1 -> Add_4dab6/1
  Divide_e5b49/1 -> Add_809c3/1
  Constant_x_qd_179db/1 -> Add_4dab6/2
  State_psi_kq_SG_D_2_69c0a/1 -> Product_80218/1
  Add_3aa3a/1 -> Subtract_cdbd8/1
  Constant_x_ddd_8ff67/1 -> Subtract_0f46b/2
  Subtract_efc4f/1 -> Product_80218/2
  Product_9cdc9/1 -> Add_6b69c/1
  Constant_x_qd_24ffc/1 -> Add_6b69c/2
  Constant_-1_d5e2f/1 -> Product_1e598/1
  Constant_x_l_4b18d/1 -> Subtract_8bd1d/2
  Constant_x_dd_1c1a3/1 -> Subtract_0f46b/1
  Product_67151/1 -> Divide_05d18/1
  Divide_859a3/1 -> Subtract_cdbd8/2
  Add_4dab6/1 -> Divide_05d18/2
  Product_f553d/1 -> Divide_7c35b/1
  Product_80218/1 -> Divide_ffc3b/1
  Constant_-1_c1860/1 -> Product_ae213/1
  Product_1e598/1 -> Product_3b575/1
  Add_6b69c/1 -> Divide_ffc3b/2
  Constant_x_dd_4b546/1 -> Subtract_01084/1
  Subtract_cdbd8/1 -> Product_f553d/1
  Subtract_ce231/1 -> Product_6aa76/2
  Constant_x_l_2477e/1 -> Subtract_01084/2
  Constant_x_ddd_15a6e/1 -> Subtract_ce231/1
  Constant_x_l_96a62/1 -> Subtract_ce231/2
  Divide_05d18/1 -> Subtract_c16dc/1
  Divide_7c35b/1 -> Add_809c3/2
  Product_6aa76/1 -> Divide_859a3/1
  Divide_ffc3b/1 -> Subtract_c16dc/2
  Subtract_8bd1d/1 -> Divide_859a3/2
  Product_3b575/1 -> Divide_99946/1
  Subtract_01084/1 -> Divide_99946/2
  Constant_x_qdd_100ca/1 -> Divide_e5b49/2
  State_psi_fd_SG_D_2_bd312/1 -> Product_6aa76/1
  Constant_x_dd_7f840/1 -> Subtract_8bd1d/1
  Subtract_c16dc/1 -> Add_424f6/1
  State_psi_q_SG_D_2_754c0/1 -> Add_424f6/2
  Constant_x_ddd_b0a16/1 -> Divide_7c35b/2
  Divide_99946/1 -> Add_3aa3a/1
  State_psi_d_SG_D_2_f9261/1 -> Add_3aa3a/2
  State_theta_SG_D_2_97c1c/1 -> MathFunc_sin_12ad6/1
  State_theta_SG_D_2_8f6ba/1 -> MathFunc_cos_e8163/1
  MathFunc_cos_e8163/1 -> Product_f553d/2
  Product_6d26f/1 -> Divide_e5b49/1
  Add_809c3/1 -> Blockout_i_q_SG_D_2_87aea/1

== system case9/Apparatus/SG_D_2/theta_SG_D_2_out_block ==
  note: theta_SG_D_2_out in case9
      | $\theta _{\mathrm{SG},D,2}$
      | Automatically generated on 2025-10-31 19:35:08 .
  State_theta_SG_D_2_ea9d6 : Inport
  Blockout_theta_SG_D_2_out_8177e : Outport
  wires:
  State_theta_SG_D_2_ea9d6/1 -> Blockout_theta_SG_D_2_out_8177e/1

== system case9/Apparatus/SG_D_2/w_SG_D_2_out_block ==
  note: w_SG_D_2_out in case9
      | $w_{\mathrm{SG},D,2}$
      | Automatically generated on 2025-10-31 19:35:08 .
  State_w_SG_D_2_5e73c : Inport
  Blockout_w_SG_D_2_out_35f1a : Outport
  wires:
  State_w_SG_D_2_5e73c/1 -> Blockout_w_SG_D_2_out_35f1a/1

== system case9/Apparatus/SG_D_3/T_e_SG_D_3_block ==
  note: T_e_SG_D_3 in case9
      | $-\frac{\psi _{d,\mathrm{SG},D,3}\,\left(\psi _{q,\mathrm{SG},D,3}+\frac{\psi _{\mathrm{gq},\mathrm{SG},D,3}\,\left(x_{l}-x_{\mathrm{qdd}}\right)}{x_{l}-x_{\mathrm{qd}}}+\frac{\psi _{\mathrm{kq},\mathrm{SG},D,3}\,\left(x_{\mathrm{qd}}-x_{\mathrm{qdd}}\right)}{x_{l}-x_{\mathrm{qd}}}\right)}{x_{\mathrm{qdd}}}-\frac{\psi _{q,\mathrm{SG},D,3}\,\left(\frac{\psi _{\mathrm{1d},\mathrm{SG},D,3}\,\left(x_{\mathrm{dd}}-x_{\mathrm{ddd}}\right)}{x_{\mathrm{dd}}-x_{l}}-\psi _{d,\mathrm{SG},D,3}+\frac{\psi _{\mathrm{fd},\mathrm{SG},D,3}\,\left(x_{\mathrm{ddd}}-x_{l}\right)}{x_{\mathrm{dd}}-x_{l}}\right)}{x_{\mathrm{ddd}}}$
      | Automatically generated on 2025-10-31 19:35:29 .
  State_psi_d_SG_D_3_512b4 : Inport
  State_psi_gq_SG_D_3_c62ee : Inport  Port=2
  State_psi_kq_SG_D_3_9fb1b : Inport  Port=3
  State_psi_q_SG_D_3_d3f4f : Inport  Port=4
  State_psi_q_SG_D_3_00123 : Inport  Port=5
  State_psi_1d_SG_D_3_9be48 : Inport  Port=6
  State_psi_d_SG_D_3_e9336 : Inport  Port=7
  State_psi_fd_SG_D_3_168b8 : Inport  Port=8
  Add_09885 : Sum
  Add_60015 : Sum
  Add_9f7c5 : Sum
  Add_a8edb : Sum
  Add_e2bec : Sum
  Add_e3544 : Sum
  Constant_-1_0a17d : Constant  Value=-1
  Constant_-1_106c4 : Constant  Value=-1
  Constant_-1_2e186 : Constant  Value=-1
  Constant_-1_45aee : Constant  Value=-1
  Constant_-1_e3141 : Constant  Value=-1
  Constant_x_dd_09bd9 : Constant  Value=x_dd
  Constant_x_dd_0f446 : Constant  Value=x_dd
  Constant_x_dd_6ea4b : Constant  Value=x_dd
  Constant_x_ddd_32c47 : Constant  Value=x_ddd
  Constant_x_ddd_44540 : Constant  Value=x_ddd
  Constant_x_ddd_e8d5e : Constant  Value=x_ddd
  Constant_x_l_091cb : Constant  Value=x_l
  Constant_x_l_97517 : Constant  Value=x_l
  Constant_x_l_b4d20 : Constant  Value=x_l
  Constant_x_l_e09c3 : Constant  Value=x_l
  Constant_x_l_ebe72 : Constant  Value=x_l
  Constant_x_l_f0323 : Constant  Value=x_l
  Constant_x_qd_08ee4 : Constant  Value=x_qd
  Constant_x_qd_251f6 : Constant  Value=x_qd
  Constant_x_qd_9d077 : Constant  Value=x_qd
  Constant_x_qdd_1a0e3 : Constant  Value=x_qdd
  Constant_x_qdd_35d45 : Constant  Value=x_qdd
  Constant_x_qdd_abdd4 : Constant  Value=x_qdd
  Divide_1060b : Product  Inputs=*/
  Divide_67357 : Product  Inputs=*/
  Divide_8157b : Product  Inputs=*/
  Divide_b933a : Product  Inputs=*/
  Divide_bfc78 : Product  Inputs=*/
  Divide_ef914 : Product  Inputs=*/
  Product_35b58 : Product
  Product_54e0e : Product
  Product_683e7 : Product
  Product_851d3 : Product
  Product_8605e : Product
  Product_a6208 : Product
  Product_b63f1 : Product
  Product_c0117 : Product
  Product_f136a : Product
  Product_f4e5a : Product
  Product_ffdf8 : Product
  Subtract_13544 : Sum  Inputs=+-
  Subtract_2a94b : Sum  Inputs=+-
  Subtract_694e3 : Sum  Inputs=+-
  Subtract_8ae9b : Sum  Inputs=+-
  Subtract_9a31b : Sum  Inputs=+-
  Subtract_d362a : Sum  Inputs=+-
  Subtract_f7fc6 : Sum  Inputs=+-
  Blockout_T_e_SG_D_3_330d1 : Outport
  wires:
  State_psi_q_SG_D_3_d3f4f/1 -> Add_e2bec/2
  Constant_-1_e3141/1 -> Product_683e7/1
  Subtract_694e3/1 -> Product_35b58/2
  State_psi_1d_SG_D_3_9be48/1 -> Product_b63f1/2
  Constant_-1_2e186/1 -> Product_54e0e/1
  Constant_x_l_091cb/1 -> Product_54e0e/2
  Add_e3544/1 -> Subtract_694e3/1
  State_psi_d_SG_D_3_e9336/1 -> Add_e3544/2
  Product_54e0e/1 -> Add_09885/1
  Constant_x_qdd_1a0e3/1 -> Subtract_d362a/2
  Add_e2bec/1 -> Product_f4e5a/2
  Constant_x_qdd_35d45/1 -> Add_09885/2
  State_psi_q_SG_D_3_00123/1 -> Product_35b58/1
  Constant_x_l_ebe72/1 -> Product_683e7/2
  Subtract_2a94b/1 -> Divide_bfc78/2
  Constant_x_l_f0323/1 -> Subtract_9a31b/2
  Constant_x_qd_08ee4/1 -> Subtract_d362a/1
  Constant_-1_0a17d/1 -> Product_a6208/1
  Subtract_f7fc6/1 -> Divide_8157b/2
  Constant_x_l_e09c3/1 -> Product_a6208/2
  Product_c0117/1 -> Divide_8157b/1
  Constant_-1_45aee/1 -> Product_b63f1/1
  Product_b63f1/1 -> Product_c0117/1
  Constant_x_dd_6ea4b/1 -> Subtract_8ae9b/1
  Constant_x_ddd_32c47/1 -> Subtract_8ae9b/2
  Add_60015/1 -> Blockout_T_e_SG_D_3_330d1/1
  State_psi_gq_SG_D_3_c62ee/1 -> Product_ffdf8/1
  Product_35b58/1 -> Divide_1060b/1
  Add_09885/1 -> Product_ffdf8/2
  State_psi_fd_SG_D_3_168b8/1 -> Product_851d3/1
  Product_683e7/1 -> Add_a8edb/1
  Constant_x_qd_251f6/1 -> Add_a8edb/2
  Constant_x_dd_0f446/1 -> Subtract_f7fc6/1
  State_psi_kq_SG_D_3_9fb1b/1 -> Product_f136a/1
  Constant_x_dd_09bd9/1 -> Subtract_2a94b/1
  Subtract_d362a/1 -> Product_f136a/2
  Product_f4e5a/1 -> Divide_67357/1
  Product_a6208/1 -> Add_9f7c5/1
  Add_a8edb/1 -> Divide_ef914/2
  Constant_x_qd_9d077/1 -> Add_9f7c5/2
  Subtract_8ae9b/1 -> Product_c0117/2
  Constant_x_l_b4d20/1 -> Subtract_f7fc6/2
  Constant_x_ddd_44540/1 -> Subtract_9a31b/1
  Product_ffdf8/1 -> Divide_ef914/1
  Product_f136a/1 -> Divide_b933a/1
  Add_9f7c5/1 -> Divide_b933a/2
  Constant_x_ddd_e8d5e/1 -> Divide_1060b/2
  Subtract_9a31b/1 -> Product_851d3/2
  Divide_ef914/1 -> Subtract_13544/1
  Constant_x_l_97517/1 -> Subtract_2a94b/2
  Divide_b933a/1 -> Subtract_13544/2
  Divide_8157b/1 -> Add_e3544/1
  Product_851d3/1 -> Divide_bfc78/1
  Constant_-1_106c4/1 -> Product_8605e/1
  State_psi_d_SG_D_3_512b4/1 -> Product_8605e/2
  Subtract_13544/1 -> Add_e2bec/1
  Divide_bfc78/1 -> Subtract_694e3/2
  Product_8605e/1 -> Product_f4e5a/1
  Constant_x_qdd_abdd4/1 -> Divide_67357/2
  Divide_67357/1 -> Add_60015/1
  Divide_1060b/1 -> Add_60015/2

== system case9/Apparatus/SG_D_3/d_E_fd_SG_D_3_block ==
  note: d_E_fd_SG_D_3 in case9
      | $\frac{V_{f,\mathrm{SG},D,3}-E_{\mathrm{fd},\mathrm{SG},D,3}\,K_{E}}{T_{E}}$
      | Automatically generated on 2025-10-31 19:35:23 .
  State_E_fd_SG_D_3_049a7 : Inport
  State_V_f_SG_D_3_753d0 : Inport  Port=2
  Add_9944c : Sum
  Constant_-1_b2ef7 : Constant  Value=-1
  Constant_K_E_82654 : Constant  Value=K_E
  Constant_T_E_e3180 : Constant  Value=T_E
  Divide_ed76d : Product  Inputs=*/
  Product_d3228 : Product
  Product_d58d1 : Product
  Blockout_d_E_fd_SG_D_3_00a24 : Outport
  wires:
  State_V_f_SG_D_3_753d0/1 -> Add_9944c/2
  Constant_-1_b2ef7/1 -> Product_d3228/1
  State_E_fd_SG_D_3_049a7/1 -> Product_d3228/2
  Constant_T_E_e3180/1 -> Divide_ed76d/2
  Product_d3228/1 -> Product_d58d1/1
  Product_d58d1/1 -> Add_9944c/1
  Constant_K_E_82654/1 -> Product_d58d1/2
  Divide_ed76d/1 -> Blockout_d_E_fd_SG_D_3_00a24/1
  Add_9944c/1 -> Divide_ed76d/1

== system case9/Apparatus/SG_D_3/d_Px_1_SG_D_3_block ==
  note: d_Px_1_SG_D_3 in case9
      | $\frac{w_{\mathrm{SG},D,3}-2\,\pi \,f_{0}}{T_{w}}-\frac{\mathrm{Px}_{1,\mathrm{SG},D,3}}{T_{w}}$
      | Automatically generated on 2025-10-31 19:35:24 .
  State_Px_1_SG_D_3_2defb : Inport
  State_w_SG_D_3_1a29d : Inport  Port=2
  Add_5e745 : Sum
  Add_9612e : Sum
  Constant_-1_b1b8c : Constant  Value=-1
  Constant_-2.0_4c00a : Constant  Value=-2.0
  Constant_T_w_9e3a2 : Constant  Value=T_w
  Constant_T_w_d2211 : Constant  Value=T_w
  Constant_f0_d9512 : Constant  Value=f0
  Constant_pi_45146 : Constant  Value=pi
  Divide_515fc : Product  Inputs=*/
  Divide_8302f : Product  Inputs=*/
  Product_20a2a : Product
  Product_79ed0 : Product
  Product_fed91 : Product
  Blockout_d_Px_1_SG_D_3_d3e56 : Outport
  wires:
  Constant_f0_d9512/1 -> Product_79ed0/2
  Constant_-1_b1b8c/1 -> Product_20a2a/1
  Constant_-2.0_4c00a/1 -> Product_fed91/1
  Constant_pi_45146/1 -> Product_fed91/2
  Product_fed91/1 -> Product_79ed0/1
  State_w_SG_D_3_1a29d/1 -> Add_9612e/2
  Divide_8302f/1 -> Add_5e745/1
  State_Px_1_SG_D_3_2defb/1 -> Product_20a2a/2
  Product_79ed0/1 -> Add_9612e/1
  Product_20a2a/1 -> Divide_8302f/1
  Constant_T_w_d2211/1 -> Divide_8302f/2
  Add_9612e/1 -> Divide_515fc/1
  Constant_T_w_9e3a2/1 -> Divide_515fc/2
  Divide_515fc/1 -> Add_5e745/2
  Add_5e745/1 -> Blockout_d_Px_1_SG_D_3_d3e56/1

== system case9/Apparatus/SG_D_3/d_Px_2_SG_D_3_block ==
  note: d_Px_2_SG_D_3 in case9
      | $\frac{\mathrm{Px}_{1,\mathrm{SG},D,3}-T_{2}\,\left(\frac{\mathrm{Px}_{1,\mathrm{SG},D,3}}{T_{w}}-\frac{w_{\mathrm{SG},D,3}-2\,\pi \,f_{0}}{T_{w}}\right)}{T_{1}}-\frac{\mathrm{Px}_{2,\mathrm{SG},D,3}}{T_{1}}$
      | Automatically generated on 2025-10-31 19:35:24 .
  State_Px_2_SG_D_3_25b38 : Inport
  State_Px_1_SG_D_3_6478a : Inport  Port=2
  State_Px_1_SG_D_3_093a8 : Inport  Port=3
  State_w_SG_D_3_8ca0a : Inport  Port=4
  Add_44ac1 : Sum
  Add_635f0 : Sum
  Add_a16cb : Sum
  Add_e4009 : Sum
  Constant_-1_4153f : Constant  Value=-1
  Constant_-1_e0252 : Constant  Value=-1
  Constant_-2.0_dc1ff : Constant  Value=-2.0
  Constant_T_1_2aad6 : Constant  Value=T_1
  Constant_T_1_622c0 : Constant  Value=T_1
  Constant_T_2_a0cf2 : Constant  Value=T_2
  Constant_T_w_363d7 : Constant  Value=T_w
  Constant_T_w_b6d57 : Constant  Value=T_w
  Constant_f0_e0965 : Constant  Value=f0
  Constant_pi_27195 : Constant  Value=pi
  Divide_0f165 : Product  Inputs=*/
  Divide_23d59 : Product  Inputs=*/
  Divide_49aa7 : Product  Inputs=*/
  Divide_e47fb : Product  Inputs=*/
  Product_0e808 : Product
  Product_10ecc : Product
  Product_233d7 : Product
  Product_85d33 : Product
  Product_d3f9b : Product
  Blockout_d_Px_2_SG_D_3_b6cd9 : Outport
  wires:
  State_Px_1_SG_D_3_093a8/1 -> Product_233d7/2
  Constant_-2.0_dc1ff/1 -> Product_85d33/1
  Constant_f0_e0965/1 -> Product_0e808/2
  Constant_pi_27195/1 -> Product_85d33/2
  Product_85d33/1 -> Product_0e808/1
  State_w_SG_D_3_8ca0a/1 -> Add_635f0/2
  Constant_-1_e0252/1 -> Product_233d7/1
  Product_0e808/1 -> Add_635f0/1
  Product_233d7/1 -> Divide_e47fb/1
  Constant_T_w_b6d57/1 -> Divide_e47fb/2
  Add_635f0/1 -> Divide_23d59/1
  Constant_T_w_363d7/1 -> Divide_23d59/2
  Divide_e47fb/1 -> Add_e4009/1
  Divide_23d59/1 -> Add_e4009/2
  Constant_T_2_a0cf2/1 -> Product_10ecc/1
  Add_e4009/1 -> Product_10ecc/2
  Constant_-1_4153f/1 -> Product_d3f9b/1
  Product_10ecc/1 -> Add_44ac1/2
  State_Px_2_SG_D_3_25b38/1 -> Product_d3f9b/2
  State_Px_1_SG_D_3_6478a/1 -> Add_44ac1/1
  Product_d3f9b/1 -> Divide_49aa7/1
  Add_a16cb/1 -> Blockout_d_Px_2_SG_D_3_b6cd9/1
  Constant_T_1_622c0/1 -> Divide_49aa7/2
  Add_44ac1/1 -> Divide_0f165/1
  Constant_T_1_2aad6/1 -> Divide_0f165/2
  Divide_49aa7/1 -> Add_a16cb/1
  Divide_0f165/1 -> Add_a16cb/2

== system case9/Apparatus/SG_D_3/d_Px_3_SG_D_3_block ==
  note: d_Px_3_SG_D_3 in case9
      | $\frac{\mathrm{Px}_{2,\mathrm{SG},D,3}+T_{4}\,\left(\frac{\mathrm{Px}_{1,\mathrm{SG},D,3}-T_{2}\,\left(\frac{\mathrm{Px}_{1,\mathrm{SG},D,3}}{T_{w}}-\frac{w_{\mathrm{SG},D,3}-2\,\pi \,f_{0}}{T_{w}}\right)}{T_{1}}-\frac{\mathrm{Px}_{2,\mathrm{SG},D,3}}{T_{1}}\right)}{T_{3}}-\frac{\mathrm{Px}_{3,\mathrm{SG},D,3}}{T_{3}}$
      | Automatically generated on 2025-10-31 19:35:25 .
  State_Px_3_SG_D_3_d7db7 : Inport
  State_Px_2_SG_D_3_174a7 : Inport  Port=2
  State_Px_2_SG_D_3_03b4c : Inport  Port=3
  State_Px_1_SG_D_3_ea1bd : Inport  Port=4
  State_Px_1_SG_D_3_0cc77 : Inport  Port=5
  State_w_SG_D_3_56bc7 : Inport  Port=6
  Add_2446c : Sum
  Add_4e0e1 : Sum
  Add_4f3f9 : Sum
  Add_795a4 : Sum
  Add_7fa34 : Sum
  Add_92f9a : Sum
  Constant_-1_2b3e3 : Constant  Value=-1
  Constant_-1_a1dc2 : Constant  Value=-1
  Constant_-1_f18bb : Constant  Value=-1
  Constant_-2.0_8d389 : Constant  Value=-2.0
  Constant_T_1_1d8be : Constant  Value=T_1
  Constant_T_1_2c146 : Constant  Value=T_1
  Constant_T_2_2f047 : Constant  Value=T_2
  Constant_T_3_58be2 : Constant  Value=T_3
  Constant_T_3_5f7d4 : Constant  Value=T_3
  Constant_T_4_c3736 : Constant  Value=T_4
  Constant_T_w_4a47f : Constant  Value=T_w
  Constant_T_w_d129c : Constant  Value=T_w
  Constant_f0_4dbf0 : Constant  Value=f0
  Constant_pi_9ea2c : Constant  Value=pi
  Divide_09951 : Product  Inputs=*/
  Divide_61ccd : Product  Inputs=*/
  Divide_c141d : Product  Inputs=*/
  Divide_dc1bb : Product  Inputs=*/
  Divide_e57ff : Product  Inputs=*/
  Divide_ee1a8 : Product  Inputs=*/
  Product_11048 : Product
  Product_22001 : Product
  Product_39ce3 : Product
  Product_54d9b : Product
  Product_69feb : Product
  Product_ce53f : Product
  Product_f6a36 : Product
  Blockout_d_Px_3_SG_D_3_3572e : Outport
  wires:
  State_Px_1_SG_D_3_0cc77/1 -> Product_69feb/2
  Constant_f0_4dbf0/1 -> Product_22001/2
  Constant_-2.0_8d389/1 -> Product_11048/1
  Add_4e0e1/1 -> Divide_dc1bb/1
  Constant_pi_9ea2c/1 -> Product_11048/2
  Product_11048/1 -> Product_22001/1
  State_w_SG_D_3_56bc7/1 -> Add_2446c/2
  Constant_T_w_4a47f/1 -> Divide_09951/2
  Constant_-1_2b3e3/1 -> Product_69feb/1
  Product_22001/1 -> Add_2446c/1
  Product_69feb/1 -> Divide_09951/1
  Add_2446c/1 -> Divide_61ccd/1
  Product_f6a36/1 -> Divide_c141d/1
  Constant_T_w_d129c/1 -> Divide_61ccd/2
  Divide_09951/1 -> Add_4f3f9/1
  Divide_61ccd/1 -> Add_4f3f9/2
  Constant_T_2_2f047/1 -> Product_39ce3/1
  Add_4f3f9/1 -> Product_39ce3/2
  Constant_-1_f18bb/1 -> Product_f6a36/1
  State_Px_2_SG_D_3_03b4c/1 -> Product_f6a36/2
  State_Px_1_SG_D_3_ea1bd/1 -> Add_4e0e1/1
  Constant_T_3_5f7d4/1 -> Divide_e57ff/2
  Product_39ce3/1 -> Add_4e0e1/2
  Constant_T_1_1d8be/1 -> Divide_c141d/2
  Add_7fa34/1 -> Product_ce53f/2
  Constant_T_1_2c146/1 -> Divide_dc1bb/2
  Divide_ee1a8/1 -> Add_92f9a/2
  Divide_c141d/1 -> Add_7fa34/1
  Divide_dc1bb/1 -> Add_7fa34/2
  Constant_T_4_c3736/1 -> Product_ce53f/1
  Constant_-1_a1dc2/1 -> Product_54d9b/1
  State_Px_3_SG_D_3_d7db7/1 -> Product_54d9b/2
  State_Px_2_SG_D_3_174a7/1 -> Add_795a4/1
  Product_ce53f/1 -> Add_795a4/2
  Product_54d9b/1 -> Divide_e57ff/1
  Add_795a4/1 -> Divide_ee1a8/1
  Constant_T_3_58be2/1 -> Divide_ee1a8/2
  Divide_e57ff/1 -> Add_92f9a/1
  Add_92f9a/1 -> Blockout_d_Px_3_SG_D_3_3572e/1
